simulink model "portail_6"  (R2016b)
settings: Solver=VariableStepAuto  StartTime=0.0  StopTime=inf  RelTol=1e-3  EnableMultiTasking=on
InitFcn:
  | load('smiData.mat')
undefined symbols (not defined in the file or in its folder): couronne_1, smiData, X, Y, Z
libraries: sm_lib x99, fl_lib x12, nesl_utility x5, elec_lib x2, realtime_pacer_lib x1
(part 3 of 3)

== system portail_6/Portail/Moteur_petit_vantail/bras_moteur_1_RIGID ==
  ReferenceFrame : sm_lib/Frames and Transforms/Reference Frame
  Solid : sm_lib/Body Elements/Solid  InertiaType=Custom  Mass=smiData.Solid(7).mass  MassUnits=kg  CenterOfMass=smiData.Solid(7).CoM  CenterOfMassUnits=mm  MomentsOfInertia=smiData.Solid(7).MoI  MomentsOfInertiaUnits=kg*mm^2  ProductsOfInertia=smiData.Solid(7).PoI  ProductsOfInertiaUnits=kg*mm^2  DensityBased=on  Density=1000  DensityUnits=kg/m^3  DoExposeReferenceFrame=on  SerializedFrames=<Frames/>  GraphicType=FromGeometry  MarkerShape=Sphere  MarkerSize=10  GraphicVisPropType=SimpleVisualProperties  GraphicDiffuseColor=smiData.Solid(7).color  GraphicSpecularColor=[0.5 0.5 0.5 1.0]  GraphicAmbientColor=[0.15 0.15 0.15 1.0]  GraphicEmissiveColor=[0.0 0.0 0.0 1.0]  GraphicShininess=75  GraphicOpacity=smiData.Solid(7).opacity  GeometryShape=FromFile  RectangleSize=[1 1]  RectangleSizeUnits=m  BrickDimensions=[1 1 1]  BrickDimensionUnits=m  CylinderRadius=1  CylinderRadiusUnits=m  CylinderLength=1  CylinderLengthUnits=m  SphereRadius=1  SphereRadiusUnits=m  EllipsoidRadii=[1 1 1]  EllipsoidRadiiUnits=m  ExtrusionCrossSection=[1 1; -1 1; -1 -1; 1 -1]  ExtrusionCrossSectionUnits=m  ExtrusionLength=1  ExtrusionLengthUnits=m  PolygonNumSides=3  PolygonOuterRadius=1  PolygonOuterRadiusUnits=m  ExtGeomFileType=STEP  ExtGeomFileName=bras moteur_Defaut_sldprt.STEP  ExtGeomFileUnits=m  RevolutionCrossSection=[1 1; 1 -1; 2 -1; 2 1]  RevolutionCrossSectionUnits=m  RevolutionExtent=Full  RevolutionAngle=180  RevolutionAngleUnits=deg
  F : PMIOPort  Port=1  Side=Left
  connections:
  ReferenceFrame/RConn1 -- Solid/RConn1 -- F/RConn1

== system portail_6/Portail/Petit_vantail/anneauext10_1_RIGID ==
  ReferenceFrame : sm_lib/Frames and Transforms/Reference Frame
  Solid : sm_lib/Body Elements/Solid  InertiaType=Custom  Mass=smiData.Solid(9).mass  MassUnits=kg  CenterOfMass=smiData.Solid(9).CoM  CenterOfMassUnits=mm  MomentsOfInertia=smiData.Solid(9).MoI  MomentsOfInertiaUnits=kg*mm^2  ProductsOfInertia=smiData.Solid(9).PoI  ProductsOfInertiaUnits=kg*mm^2  DensityBased=on  Density=1000  DensityUnits=kg/m^3  DoExposeReferenceFrame=on  SerializedFrames=<Frames/>  GraphicType=FromGeometry  MarkerShape=Sphere  MarkerSize=10  GraphicVisPropType=SimpleVisualProperties  GraphicDiffuseColor=smiData.Solid(9).color  GraphicSpecularColor=[0.5 0.5 0.5 1.0]  GraphicAmbientColor=[0.15 0.15 0.15 1.0]  GraphicEmissiveColor=[0.0 0.0 0.0 1.0]  GraphicShininess=75  GraphicOpacity=smiData.Solid(9).opacity  GeometryShape=FromFile  RectangleSize=[1 1]  RectangleSizeUnits=m  BrickDimensions=[1 1 1]  BrickDimensionUnits=m  CylinderRadius=1  CylinderRadiusUnits=m  CylinderLength=1  CylinderLengthUnits=m  SphereRadius=1  SphereRadiusUnits=m  EllipsoidRadii=[1 1 1]  EllipsoidRadiiUnits=m  ExtrusionCrossSection=[1 1; -1 1; -1 -1; 1 -1]  ExtrusionCrossSectionUnits=m  ExtrusionLength=1  ExtrusionLengthUnits=m  PolygonNumSides=3  PolygonOuterRadius=1  PolygonOuterRadiusUnits=m  ExtGeomFileType=STEP  ExtGeomFileName=anneauext10_Defaut_sldprt.STEP  ExtGeomFileUnits=m  RevolutionCrossSection=[1 1; 1 -1; 2 -1; 2 1]  RevolutionCrossSectionUnits=m  RevolutionExtent=Full  RevolutionAngle=180  RevolutionAngleUnits=deg
  F : PMIOPort  Port=1  Side=Left
  connections:
  ReferenceFrame/RConn1 -- Solid/RConn1 -- F/RConn1

== system portail_6/Portail/Petit_vantail/axe_chape_1_RIGID ==
  ReferenceFrame : sm_lib/Frames and Transforms/Reference Frame
  Solid : sm_lib/Body Elements/Solid  InertiaType=Custom  Mass=smiData.Solid(10).mass  MassUnits=kg  CenterOfMass=smiData.Solid(10).CoM  CenterOfMassUnits=mm  MomentsOfInertia=smiData.Solid(10).MoI  MomentsOfInertiaUnits=kg*mm^2  ProductsOfInertia=smiData.Solid(10).PoI  ProductsOfInertiaUnits=kg*mm^2  DensityBased=on  Density=1000  DensityUnits=kg/m^3  DoExposeReferenceFrame=on  SerializedFrames=<Frames/>  GraphicType=FromGeometry  MarkerShape=Sphere  MarkerSize=10  GraphicVisPropType=SimpleVisualProperties  GraphicDiffuseColor=smiData.Solid(10).color  GraphicSpecularColor=[0.5 0.5 0.5 1.0]  GraphicAmbientColor=[0.15 0.15 0.15 1.0]  GraphicEmissiveColor=[0.0 0.0 0.0 1.0]  GraphicShininess=75  GraphicOpacity=smiData.Solid(10).opacity  GeometryShape=FromFile  RectangleSize=[1 1]  RectangleSizeUnits=m  BrickDimensions=[1 1 1]  BrickDimensionUnits=m  CylinderRadius=1  CylinderRadiusUnits=m  CylinderLength=1  CylinderLengthUnits=m  SphereRadius=1  SphereRadiusUnits=m  EllipsoidRadii=[1 1 1]  EllipsoidRadiiUnits=m  ExtrusionCrossSection=[1 1; -1 1; -1 -1; 1 -1]  ExtrusionCrossSectionUnits=m  ExtrusionLength=1  ExtrusionLengthUnits=m  PolygonNumSides=3  PolygonOuterRadius=1  PolygonOuterRadiusUnits=m  ExtGeomFileType=STEP  ExtGeomFileName=axe chape_Defaut_sldprt.STEP  ExtGeomFileUnits=m  RevolutionCrossSection=[1 1; 1 -1; 2 -1; 2 1]  RevolutionCrossSectionUnits=m  RevolutionExtent=Full  RevolutionAngle=180  RevolutionAngleUnits=deg
  F : PMIOPort  Port=1  Side=Left
  connections:
  ReferenceFrame/RConn1 -- Solid/RConn1 -- F/RConn1

== system portail_6/Portail/Petit_vantail/chape_1_RIGID ==
  ReferenceFrame : sm_lib/Frames and Transforms/Reference Frame
  Solid : sm_lib/Body Elements/Solid  InertiaType=Custom  Mass=smiData.Solid(12).mass  MassUnits=kg  CenterOfMass=smiData.Solid(12).CoM  CenterOfMassUnits=mm  MomentsOfInertia=smiData.Solid(12).MoI  MomentsOfInertiaUnits=kg*mm^2  ProductsOfInertia=smiData.Solid(12).PoI  ProductsOfInertiaUnits=kg*mm^2  DensityBased=on  Density=1000  DensityUnits=kg/m^3  DoExposeReferenceFrame=on  SerializedFrames=<Frames/>  GraphicType=FromGeometry  MarkerShape=Sphere  MarkerSize=10  GraphicVisPropType=SimpleVisualProperties  GraphicDiffuseColor=smiData.Solid(12).color  GraphicSpecularColor=[0.5 0.5 0.5 1.0]  GraphicAmbientColor=[0.15 0.15 0.15 1.0]  GraphicEmissiveColor=[0.0 0.0 0.0 1.0]  GraphicShininess=75  GraphicOpacity=smiData.Solid(12).opacity  GeometryShape=FromFile  RectangleSize=[1 1]  RectangleSizeUnits=m  BrickDimensions=[1 1 1]  BrickDimensionUnits=m  CylinderRadius=1  CylinderRadiusUnits=m  CylinderLength=1  CylinderLengthUnits=m  SphereRadius=1  SphereRadiusUnits=m  EllipsoidRadii=[1 1 1]  EllipsoidRadiiUnits=m  ExtrusionCrossSection=[1 1; -1 1; -1 -1; 1 -1]  ExtrusionCrossSectionUnits=m  ExtrusionLength=1  ExtrusionLengthUnits=m  PolygonNumSides=3  PolygonOuterRadius=1  PolygonOuterRadiusUnits=m  ExtGeomFileType=STEP  ExtGeomFileName=chape_Defaut_sldprt.STEP  ExtGeomFileUnits=m  RevolutionCrossSection=[1 1; 1 -1; 2 -1; 2 1]  RevolutionCrossSectionUnits=m  RevolutionExtent=Full  RevolutionAngle=180  RevolutionAngleUnits=deg
  F : PMIOPort  Port=1  Side=Left
  connections:
  ReferenceFrame/RConn1 -- Solid/RConn1 -- F/RConn1

== system portail_6/Portail/Petit_vantail/petit_Vantail_1_RIGID ==
  ReferenceFrame : sm_lib/Frames and Transforms/Reference Frame
  Solid : sm_lib/Body Elements/Solid  InertiaType=Custom  Mass=smiData.Solid(11).mass  MassUnits=kg  CenterOfMass=smiData.Solid(11).CoM  CenterOfMassUnits=mm  MomentsOfInertia=smiData.Solid(11).MoI  MomentsOfInertiaUnits=kg*mm^2  ProductsOfInertia=smiData.Solid(11).PoI  ProductsOfInertiaUnits=kg*mm^2  DensityBased=on  Density=1000  DensityUnits=kg/m^3  DoExposeReferenceFrame=on  SerializedFrames=<Frames/>  GraphicType=FromGeometry  MarkerShape=Sphere  MarkerSize=10  GraphicVisPropType=SimpleVisualProperties  GraphicDiffuseColor=smiData.Solid(11).color  GraphicSpecularColor=[0.5 0.5 0.5 1.0]  GraphicAmbientColor=[0.15 0.15 0.15 1.0]  GraphicEmissiveColor=[0.0 0.0 0.0 1.0]  GraphicShininess=75  GraphicOpacity=smiData.Solid(11).opacity  GeometryShape=FromFile  RectangleSize=[1 1]  RectangleSizeUnits=m  BrickDimensions=[1 1 1]  BrickDimensionUnits=m  CylinderRadius=1  CylinderRadiusUnits=m  CylinderLength=1  CylinderLengthUnits=m  SphereRadius=1  SphereRadiusUnits=m  EllipsoidRadii=[1 1 1]  EllipsoidRadiiUnits=m  ExtrusionCrossSection=[1 1; -1 1; -1 -1; 1 -1]  ExtrusionCrossSectionUnits=m  ExtrusionLength=1  ExtrusionLengthUnits=m  PolygonNumSides=3  PolygonOuterRadius=1  PolygonOuterRadiusUnits=m  ExtGeomFileType=STEP  ExtGeomFileName=petit_Vantail_Defaut_sldprt.STEP  ExtGeomFileUnits=m  RevolutionCrossSection=[1 1; 1 -1; 2 -1; 2 1]  RevolutionCrossSectionUnits=m  RevolutionExtent=Full  RevolutionAngle=180  RevolutionAngleUnits=deg
  F : PMIOPort  Port=1  Side=Left
  connections:
  ReferenceFrame/RConn1 -- Solid/RConn1 -- F/RConn1

== stateflow chart portail_6/acquisition clavier/Chart1 ==
  state depart
  state etape1
  state etape2
  state etape3
  state etape4
    entry:clavier=1
    exit:clavier=0
  (default) -> depart
  etape2 -> etape3 : [touche3==1]
  etape3 -> etape4 : [touche4==1]
  etape1 -> etape2 : [touche2==1]
  depart -> etape1 : [touche1==1]
  etape4 -> depart : after(1,sec)
  data: touche1 input; touche2 input; touche3 input; touche4 input; clavier output; touche5 input; touche6 input; touche7 input; touche8 input; touche9 input; touche0 input

== stateflow chart portail_6/Chart ==
  state moteur_petit_vantail [parallel]
    settings: executionOrder=2
    state rotation_positive_pv
      entry:marche_mpv=1,sens_mpv=1
    state arret_pv
      entry:marche_mpv=0
    state Attente
    state rotation_negative_pv
      entry:marche_mpv=1,sens_mpv=-1
    rotation_positive_pv -> arret_pv : [(fdc_ouvert_pv==1||teleco==1)&&after(0.5,sec)]
    arret_pv -> rotation_positive_pv [order 1] : [(teleco==1||clavier==1)&&fdc_ouvert_pv==0]
    rotation_negative_pv -> rotation_positive_pv [order 2] : [cellule==1]
    (default) -> arret_pv
    rotation_negative_pv -> arret_pv [order 1] : [(teleco==1||fdc_ferme_pv==1)&&after(0.5,sec)]
    arret_pv -> moteur_petit_vantail.Attente [order 2] : [teleco==1&&fdc_ouvert_pv==1&&cellule==0]
    moteur_petit_vantail.Attente -> rotation_negative_pv : [after(1,sec)&&in(moteur_grand_vantail.rotation_negative_gv)]
  state moteur_grand_vantail [parallel]
    settings: executionOrder=1
    state rotation_positive_gv
      entry:marche_mgv=1,sens_mgv=1
    state Attente
    state arret_gv
      entry:marche_mgv=0
    state rotation_negative_gv
      entry:marche_mgv=1,sens_mgv=-1
    rotation_positive_gv -> arret_gv : [(fdc_ouvert_gv==1||teleco==1)&&after(0.5,sec)]
    moteur_grand_vantail.Attente -> rotation_positive_gv : [after(1,sec)&&in(moteur_petit_vantail.rotation_positive_pv)]
    rotation_negative_gv -> rotation_positive_gv [order 2] : [cellule==1]
    arret_gv -> moteur_grand_vantail.Attente [order 1] : [(teleco==1||clavier==1)&&fdc_ouvert_gv==0]
    (default) -> arret_gv
    arret_gv -> rotation_negative_gv [order 2] : [teleco==1&&fdc_ouvert_gv==1&&cellule==0]
    rotation_negative_gv -> arret_gv [order 1] : [(teleco==1||fdc_ferme_gv==1)&&after(0.5,sec)]
  state gestion_fin_de_course_pv [parallel]
    settings: executionOrder=3
    state depart
      entry:fdc_ouvert_pv=0,fdc_ferme_pv=1
    state pv_ouvert
      entry:fdc_ouvert_pv=1
    state pv_plus_ferme
      entry:fdc_ferme_pv=0
    state plus_ouvert
      entry:fdc_ouvert_pv=0
    (default) -> gestion_fin_de_course_pv.depart
    gestion_fin_de_course_pv.depart -> pv_plus_ferme : [position_petit_vantail>1]
    pv_plus_ferme -> pv_ouvert [order 1] : [position_petit_vantail>89]
    pv_plus_ferme -> gestion_fin_de_course_pv.depart [order 2] : [position_petit_vantail<1]
    gestion_fin_de_course_pv.plus_ouvert -> gestion_fin_de_course_pv.depart [order 1] : [position_petit_vantail<1]
    gestion_fin_de_course_pv.plus_ouvert -> pv_ouvert [order 2] : [position_petit_vantail>89]
    pv_ouvert -> gestion_fin_de_course_pv.plus_ouvert : [position_petit_vantail<89]
  state gestion_fin_de_course_gv [parallel]
    settings: executionOrder=4
    state depart
      entry:fdc_ouvert_gv=0,fdc_ferme_gv=1
    state gv_ouvert
      entry:fdc_ouvert_gv=1
    state gv_plus_ferme
      entry:fdc_ferme_gv=0
    state plus_ouvert
      entry:fdc_ouvert_gv=0
    (default) -> gestion_fin_de_course_gv.depart
    gestion_fin_de_course_gv.depart -> gv_plus_ferme : [position_grand_vantail>1]
    gv_plus_ferme -> gv_ouvert [order 1] : [position_grand_vantail>89]
    gv_plus_ferme -> gestion_fin_de_course_gv.depart [order 2] : [position_grand_vantail<1]
    gestion_fin_de_course_gv.plus_ouvert -> gv_ouvert [order 2] : [position_grand_vantail>89]
    gv_ouvert -> gestion_fin_de_course_gv.plus_ouvert : [position_grand_vantail<89]
    gestion_fin_de_course_gv.plus_ouvert -> gestion_fin_de_course_gv.depart [order 1] : [position_grand_vantail<1]
  data: clavier input; marche_mpv output; marche_mgv output; sens_mgv output; sens_mpv output; teleco input; cellule input; position_petit_vantail input; fdc_ferme_pv local; fdc_ouvert_pv local; position_grand_vantail input; fdc_ouvert_gv local; fdc_ferme_gv local
